simulink model "lat_ailInput"  (R2016a)
settings: Solver=VariableStepAuto  StartTime=0.0  StopTime=200  RelTol=1e-3
undefined symbols (not defined in the file): Alat, Blat, Clat, Dlat
settings Model: Creator=Gray  LastModifiedBy=Gray

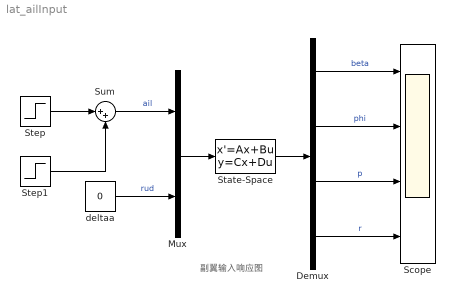
== system lat_ailInput ==
  note: 副翼输入响应图
  Demux : Demux
  Mux : Mux  Inputs=2
  Scope : Scope  NumInputPorts=4
  State-Space : StateSpace  A=Alat  B=Blat  C=Clat  D=Dlat  X0="[0  0 0 0]'"
  Step : Step  After=2  SampleTime=0
  Step1 : Step  Time=2  After=-2  SampleTime=0
  Sum : Sum  Inputs=|++
  deltaa : Constant  Value=0
  wires:
  State-Space/1 -> Demux/1
  Mux/1 -> State-Space/1
  Demux/1 -> Scope/1  "beta"
  Demux/2 -> Scope/2  "phi"
  Demux/3 -> Scope/3  "p"
  Demux/4 -> Scope/4  "r"
  Step/1 -> Sum/1
  Step1/1 -> Sum/2
  Sum/1 -> Mux/1  "ail"
  deltaa/1 -> Mux/2  "rud"
